simulink library "SendToSOMANET"  (R2016b)
settings: Solver=VariableStepAuto  StartTime=0.0  StopTime=10.0  RelTol=1e-3
undefined symbols (not defined in the file): jointPolarityLHFE, jointPolarityLKFE, jointPolarityRHFE, jointPolarityRKFE, resolutionJointEncoder, torquePolarityLHFE, torquePolarityLKFE, torquePolarityRHFE, torquePolarityRKFE, zeroOffsetLHFE, zeroOffsetLKFE, zeroOffsetRHFE, zeroOffsetRKFE
libraries: xpcethercatlib x35, ConversionsLibrary x32, simulink_extras x8
settings Model: Creator=Nathan  LastModifiedBy=march

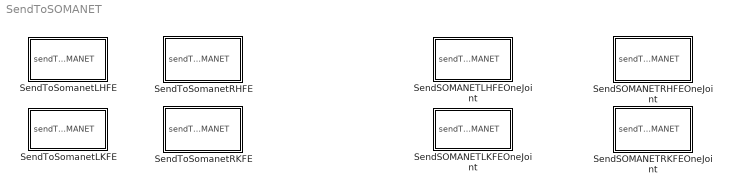
== system SendToSOMANET ==
  SendSOMANETLHFEOneJoint : Subsystem
  SendSOMANETLKFEOneJoint : Subsystem
  SendSOMANETRHFEOneJoint : Subsystem
  SendSOMANETRKFEOneJoint : Subsystem
  SendToSomanetLHFE : Subsystem
  SendToSomanetLKFE : Subsystem
  SendToSomanetRHFE : Subsystem
  SendToSomanetRKFE : Subsystem

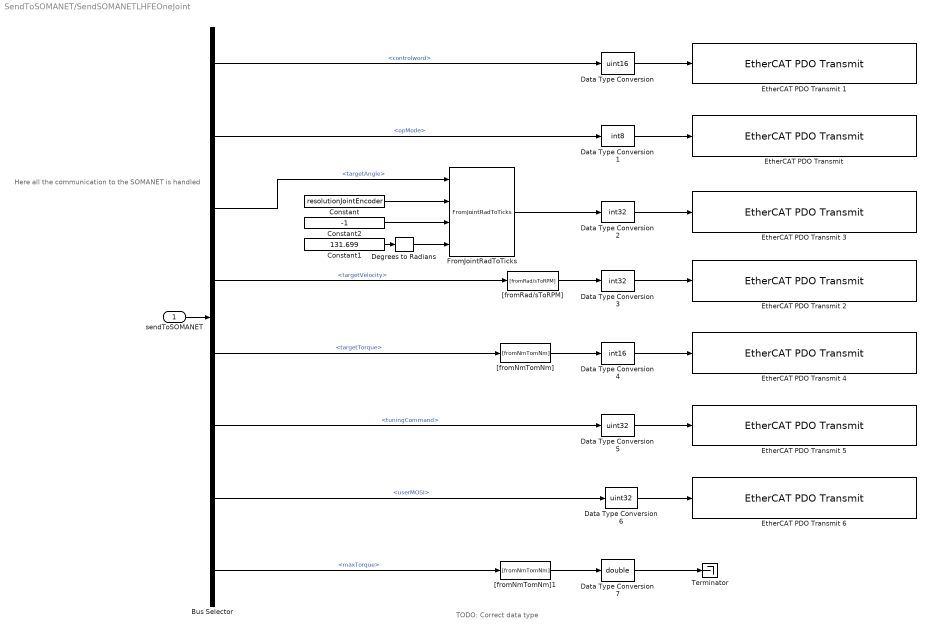
== system SendToSOMANET/SendSOMANETLHFEOneJoint ==
  note: Here all the communication to the SOMANET is handled
  note: TODO: Correct data type
  sendToSOMANET : Inport  OutDataTypeStr=Bus: EtherCATSendToSOMANET  BusOutputAsStruct=on
  Bus Selector : BusSelector  OutputSignals=controlword,opMode,targetAngle,targetVelocity,targetTorque,tuningCommand,userMOSI,maxTorque
  Constant : Constant  Value=resolutionJointEncoder
  Constant1 : Constant  Value=131.699  SampleTime=-1
  Constant2 : Constant  Value=-1
  Data Type Conversion : DataTypeConversion  OutDataTypeStr=uint16  RndMeth=Nearest
  Data Type Conversion1 : DataTypeConversion  OutDataTypeStr=int8  RndMeth=Nearest
  Data Type Conversion2 : DataTypeConversion  OutDataTypeStr=int32  RndMeth=Nearest
  Data Type Conversion3 : DataTypeConversion  OutDataTypeStr=int32  RndMeth=Nearest
  Data Type Conversion4 : DataTypeConversion  OutDataTypeStr=int16  RndMeth=Nearest
  Data Type Conversion5 : DataTypeConversion  OutDataTypeStr=uint32  RndMeth=Nearest
  Data Type Conversion6 : DataTypeConversion  OutDataTypeStr=uint32  RndMeth=Nearest
  Data Type Conversion7 : DataTypeConversion  OutDataTypeStr=double  RndMeth=Nearest
  Degrees to Radians : simulink_extras/Transformations/Degrees to Radians
  "EtherCAT PDO Transmit " : xpcethercatlib/EtherCAT PDO Transmit   Priority=3  sig_name=Drive 1 LHFE.Outputs.Op Mode  sig_offset=224  sig_type=int8  type_size=8  sig_dim=1  device_id=0  sample_time=0.002000
  EtherCAT PDO Transmit 1 : xpcethercatlib/EtherCAT PDO Transmit   Priority=3  sig_name=Drive 1 LHFE.Outputs.Controlword  sig_offset=208  sig_type=uint16  type_size=16  sig_dim=1  device_id=0  sample_time=0.002000
  EtherCAT PDO Transmit 2 : xpcethercatlib/EtherCAT PDO Transmit   Priority=3  sig_name=Drive 1 LHFE.Outputs.Target Velocity  sig_offset=280  sig_type=int32  type_size=32  sig_dim=1  device_id=0  sample_time=0.002000
  EtherCAT PDO Transmit 3 : xpcethercatlib/EtherCAT PDO Transmit   Priority=3  sig_name=Drive 1 LHFE.Outputs.Target Position  sig_offset=248  sig_type=int32  type_size=32  sig_dim=1  device_id=0  sample_time=0.002000
  EtherCAT PDO Transmit 4 : xpcethercatlib/EtherCAT PDO Transmit   Priority=3  sig_name=Drive 1 LHFE.Outputs.Target Torque  sig_offset=232  sig_type=int16  type_size=16  sig_dim=1  device_id=0  sample_time=0.002000
  EtherCAT PDO Transmit 5 : xpcethercatlib/EtherCAT PDO Transmit   Priority=3  sig_name=Drive 1 LHFE.Outputs.Tuning command  sig_offset=344  sig_type=uint32  type_size=32  sig_dim=1  device_id=0  sample_time=0.002000
  EtherCAT PDO Transmit 6 : xpcethercatlib/EtherCAT PDO Transmit   Priority=3  sig_name=Drive 1 LHFE.Outputs.User MOSI  sig_offset=408  sig_type=uint32  type_size=32  sig_dim=1  device_id=0  sample_time=0.002000
  FromJointRadToTicks : ConversionsLibrary/FromJointRadToTicks
  Terminator : Terminator
  "[fromNmTomNm]" : ConversionsLibrary/[fromNmTomNm]
  "[fromNmTomNm]1" : ConversionsLibrary/[fromNmTomNm]
  "[fromRad/sToRPM]" : ConversionsLibrary/[fromRad//sToRPM]
  wires:
  Bus Selector/1 -> Data Type Conversion/1  "<controlword>"
  "[fromRad/sToRPM]"/1 -> Data Type Conversion3/1
  Bus Selector/7 -> Data Type Conversion6/1  "<userMOSI>"
  Bus Selector/8 -> "[fromNmTomNm]1"/1  "<maxTorque>"
  Bus Selector/4 -> "[fromRad/sToRPM]"/1  "<targetVelocity>"
  "[fromNmTomNm]1"/1 -> Data Type Conversion7/1
  "[fromNmTomNm]"/1 -> Data Type Conversion4/1
  Bus Selector/6 -> Data Type Conversion5/1  "<tuningCommand>"
  Bus Selector/2 -> Data Type Conversion1/1  "<opMode>"
  Bus Selector/5 -> "[fromNmTomNm]"/1  "<targetTorque>"
  Data Type Conversion/1 -> EtherCAT PDO Transmit 1/1
  Data Type Conversion4/1 -> EtherCAT PDO Transmit 4/1
  Data Type Conversion3/1 -> EtherCAT PDO Transmit 2/1
  Data Type Conversion2/1 -> EtherCAT PDO Transmit 3/1
  Data Type Conversion1/1 -> "EtherCAT PDO Transmit "/1
  Data Type Conversion5/1 -> EtherCAT PDO Transmit 5/1
  Data Type Conversion6/1 -> EtherCAT PDO Transmit 6/1
  Data Type Conversion7/1 -> Terminator/1
  sendToSOMANET/1 -> Bus Selector/1
  Constant1/1 -> Degrees to Radians/1
  Bus Selector/3 -> FromJointRadToTicks/1  "<targetAngle>"
  Degrees to Radians/1 -> FromJointRadToTicks/4
  Constant/1 -> FromJointRadToTicks/2
  Constant2/1 -> FromJointRadToTicks/3
  FromJointRadToTicks/1 -> Data Type Conversion2/1

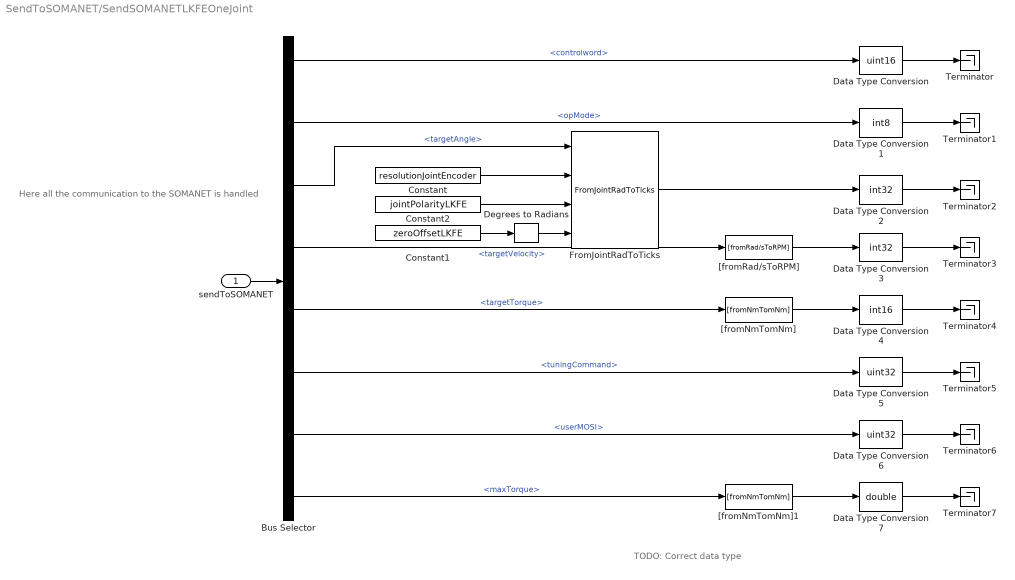
== system SendToSOMANET/SendSOMANETLKFEOneJoint ==
  note: Here all the communication to the SOMANET is handled
  note: TODO: Correct data type
  sendToSOMANET : Inport  OutDataTypeStr=Bus: EtherCATSendToSOMANET  BusOutputAsStruct=on
  Bus Selector : BusSelector  OutputSignals=controlword,opMode,targetAngle,targetVelocity,targetTorque,tuningCommand,userMOSI,maxTorque
  Constant : Constant  Value=resolutionJointEncoder
  Constant1 : Constant  Value=zeroOffsetLKFE  SampleTime=-1
  Constant2 : Constant  Value=jointPolarityLKFE
  Data Type Conversion : DataTypeConversion  OutDataTypeStr=uint16  RndMeth=Nearest
  Data Type Conversion1 : DataTypeConversion  OutDataTypeStr=int8  RndMeth=Nearest
  Data Type Conversion2 : DataTypeConversion  OutDataTypeStr=int32  RndMeth=Nearest
  Data Type Conversion3 : DataTypeConversion  OutDataTypeStr=int32  RndMeth=Nearest
  Data Type Conversion4 : DataTypeConversion  OutDataTypeStr=int16  RndMeth=Nearest
  Data Type Conversion5 : DataTypeConversion  OutDataTypeStr=uint32  RndMeth=Nearest
  Data Type Conversion6 : DataTypeConversion  OutDataTypeStr=uint32  RndMeth=Nearest
  Data Type Conversion7 : DataTypeConversion  OutDataTypeStr=double  RndMeth=Nearest
  Degrees to Radians : simulink_extras/Transformations/Degrees to Radians
  FromJointRadToTicks : ConversionsLibrary/FromJointRadToTicks
  Terminator{,1..7} (8 alike) : Terminator
  "[fromNmTomNm]" : ConversionsLibrary/[fromNmTomNm]
  "[fromNmTomNm]1" : ConversionsLibrary/[fromNmTomNm]
  "[fromRad/sToRPM]" : ConversionsLibrary/[fromRad//sToRPM]
  wires:
  Bus Selector/1 -> Data Type Conversion/1  "<controlword>"
  "[fromRad/sToRPM]"/1 -> Data Type Conversion3/1
  Bus Selector/7 -> Data Type Conversion6/1  "<userMOSI>"
  Bus Selector/8 -> "[fromNmTomNm]1"/1  "<maxTorque>"
  "[fromNmTomNm]1"/1 -> Data Type Conversion7/1
  "[fromNmTomNm]"/1 -> Data Type Conversion4/1
  Bus Selector/6 -> Data Type Conversion5/1  "<tuningCommand>"
  Bus Selector/2 -> Data Type Conversion1/1  "<opMode>"
  sendToSOMANET/1 -> Bus Selector/1
  Bus Selector/5 -> "[fromNmTomNm]"/1  "<targetTorque>"
  Data Type Conversion/1 -> Terminator/1
  Data Type Conversion1/1 -> Terminator1/1
  Data Type Conversion2/1 -> Terminator2/1
  Data Type Conversion3/1 -> Terminator3/1
  Data Type Conversion4/1 -> Terminator4/1
  Data Type Conversion5/1 -> Terminator5/1
  Data Type Conversion6/1 -> Terminator6/1
  Data Type Conversion7/1 -> Terminator7/1
  Bus Selector/3 -> FromJointRadToTicks/1  "<targetAngle>"
  Constant/1 -> FromJointRadToTicks/2
  Constant2/1 -> FromJointRadToTicks/3
  FromJointRadToTicks/1 -> Data Type Conversion2/1
  Constant1/1 -> Degrees to Radians/1
  Degrees to Radians/1 -> FromJointRadToTicks/4
  Bus Selector/4 -> "[fromRad/sToRPM]"/1  "<targetVelocity>"

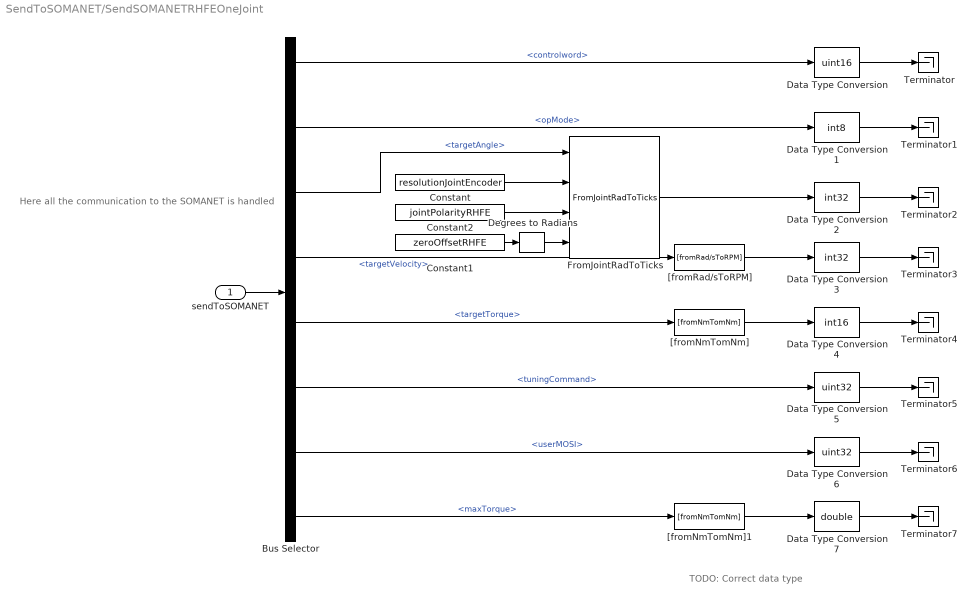
== system SendToSOMANET/SendSOMANETRHFEOneJoint ==
  note: Here all the communication to the SOMANET is handled
  note: TODO: Correct data type
  sendToSOMANET : Inport  OutDataTypeStr=Bus: EtherCATSendToSOMANET  BusOutputAsStruct=on
  Bus Selector : BusSelector  OutputSignals=controlword,opMode,targetAngle,targetVelocity,targetTorque,tuningCommand,userMOSI,maxTorque
  Constant : Constant  Value=resolutionJointEncoder
  Constant1 : Constant  Value=zeroOffsetRHFE  SampleTime=-1
  Constant2 : Constant  Value=jointPolarityRHFE
  Data Type Conversion : DataTypeConversion  OutDataTypeStr=uint16  RndMeth=Nearest
  Data Type Conversion1 : DataTypeConversion  OutDataTypeStr=int8  RndMeth=Nearest
  Data Type Conversion2 : DataTypeConversion  OutDataTypeStr=int32  RndMeth=Nearest
  Data Type Conversion3 : DataTypeConversion  OutDataTypeStr=int32  RndMeth=Nearest
  Data Type Conversion4 : DataTypeConversion  OutDataTypeStr=int16  RndMeth=Nearest
  Data Type Conversion5 : DataTypeConversion  OutDataTypeStr=uint32  RndMeth=Nearest
  Data Type Conversion6 : DataTypeConversion  OutDataTypeStr=uint32  RndMeth=Nearest
  Data Type Conversion7 : DataTypeConversion  OutDataTypeStr=double  RndMeth=Nearest
  Degrees to Radians : simulink_extras/Transformations/Degrees to Radians
  FromJointRadToTicks : ConversionsLibrary/FromJointRadToTicks
  Terminator{,1..7} (8 alike) : Terminator
  "[fromNmTomNm]" : ConversionsLibrary/[fromNmTomNm]
  "[fromNmTomNm]1" : ConversionsLibrary/[fromNmTomNm]
  "[fromRad/sToRPM]" : ConversionsLibrary/[fromRad//sToRPM]
  wires:
  Bus Selector/1 -> Data Type Conversion/1  "<controlword>"
  "[fromRad/sToRPM]"/1 -> Data Type Conversion3/1
  Bus Selector/7 -> Data Type Conversion6/1  "<userMOSI>"
  Bus Selector/8 -> "[fromNmTomNm]1"/1  "<maxTorque>"
  "[fromNmTomNm]1"/1 -> Data Type Conversion7/1
  "[fromNmTomNm]"/1 -> Data Type Conversion4/1
  Bus Selector/6 -> Data Type Conversion5/1  "<tuningCommand>"
  Bus Selector/2 -> Data Type Conversion1/1  "<opMode>"
  sendToSOMANET/1 -> Bus Selector/1
  Bus Selector/5 -> "[fromNmTomNm]"/1  "<targetTorque>"
  Data Type Conversion/1 -> Terminator/1
  Data Type Conversion1/1 -> Terminator1/1
  Data Type Conversion2/1 -> Terminator2/1
  Data Type Conversion3/1 -> Terminator3/1
  Data Type Conversion4/1 -> Terminator4/1
  Data Type Conversion5/1 -> Terminator5/1
  Data Type Conversion6/1 -> Terminator6/1
  Data Type Conversion7/1 -> Terminator7/1
  Bus Selector/3 -> FromJointRadToTicks/1  "<targetAngle>"
  Constant/1 -> FromJointRadToTicks/2
  Constant2/1 -> FromJointRadToTicks/3
  FromJointRadToTicks/1 -> Data Type Conversion2/1
  Constant1/1 -> Degrees to Radians/1
  Degrees to Radians/1 -> FromJointRadToTicks/4
  Bus Selector/4 -> "[fromRad/sToRPM]"/1  "<targetVelocity>"

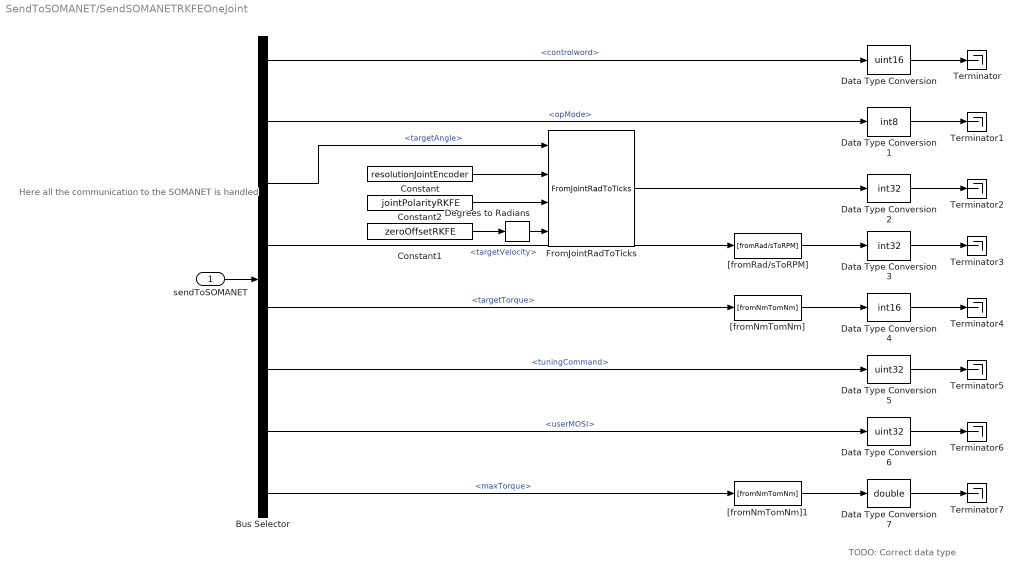
== system SendToSOMANET/SendSOMANETRKFEOneJoint ==
  note: Here all the communication to the SOMANET is handled
  note: TODO: Correct data type
  sendToSOMANET : Inport  OutDataTypeStr=Bus: EtherCATSendToSOMANET  BusOutputAsStruct=on
  Bus Selector : BusSelector  OutputSignals=controlword,opMode,targetAngle,targetVelocity,targetTorque,tuningCommand,userMOSI,maxTorque
  Constant : Constant  Value=resolutionJointEncoder
  Constant1 : Constant  Value=zeroOffsetRKFE  SampleTime=-1
  Constant2 : Constant  Value=jointPolarityRKFE
  Data Type Conversion : DataTypeConversion  OutDataTypeStr=uint16  RndMeth=Nearest
  Data Type Conversion1 : DataTypeConversion  OutDataTypeStr=int8  RndMeth=Nearest
  Data Type Conversion2 : DataTypeConversion  OutDataTypeStr=int32  RndMeth=Nearest
  Data Type Conversion3 : DataTypeConversion  OutDataTypeStr=int32  RndMeth=Nearest
  Data Type Conversion4 : DataTypeConversion  OutDataTypeStr=int16  RndMeth=Nearest
  Data Type Conversion5 : DataTypeConversion  OutDataTypeStr=uint32  RndMeth=Nearest
  Data Type Conversion6 : DataTypeConversion  OutDataTypeStr=uint32  RndMeth=Nearest
  Data Type Conversion7 : DataTypeConversion  OutDataTypeStr=double  RndMeth=Nearest
  Degrees to Radians : simulink_extras/Transformations/Degrees to Radians
  FromJointRadToTicks : ConversionsLibrary/FromJointRadToTicks
  Terminator{,1..7} (8 alike) : Terminator
  "[fromNmTomNm]" : ConversionsLibrary/[fromNmTomNm]
  "[fromNmTomNm]1" : ConversionsLibrary/[fromNmTomNm]
  "[fromRad/sToRPM]" : ConversionsLibrary/[fromRad//sToRPM]
  wires:
  Bus Selector/1 -> Data Type Conversion/1  "<controlword>"
  "[fromRad/sToRPM]"/1 -> Data Type Conversion3/1
  Bus Selector/7 -> Data Type Conversion6/1  "<userMOSI>"
  Bus Selector/8 -> "[fromNmTomNm]1"/1  "<maxTorque>"
  Bus Selector/4 -> "[fromRad/sToRPM]"/1  "<targetVelocity>"
  "[fromNmTomNm]1"/1 -> Data Type Conversion7/1
  "[fromNmTomNm]"/1 -> Data Type Conversion4/1
  Bus Selector/6 -> Data Type Conversion5/1  "<tuningCommand>"
  Bus Selector/2 -> Data Type Conversion1/1  "<opMode>"
  sendToSOMANET/1 -> Bus Selector/1
  Bus Selector/5 -> "[fromNmTomNm]"/1  "<targetTorque>"
  Data Type Conversion/1 -> Terminator/1
  Data Type Conversion1/1 -> Terminator1/1
  Data Type Conversion2/1 -> Terminator2/1
  Data Type Conversion3/1 -> Terminator3/1
  Data Type Conversion4/1 -> Terminator4/1
  Data Type Conversion5/1 -> Terminator5/1
  Data Type Conversion6/1 -> Terminator6/1
  Data Type Conversion7/1 -> Terminator7/1
  Constant1/1 -> Degrees to Radians/1
  Bus Selector/3 -> FromJointRadToTicks/1  "<targetAngle>"
  Degrees to Radians/1 -> FromJointRadToTicks/4
  Constant/1 -> FromJointRadToTicks/2
  Constant2/1 -> FromJointRadToTicks/3
  FromJointRadToTicks/1 -> Data Type Conversion2/1

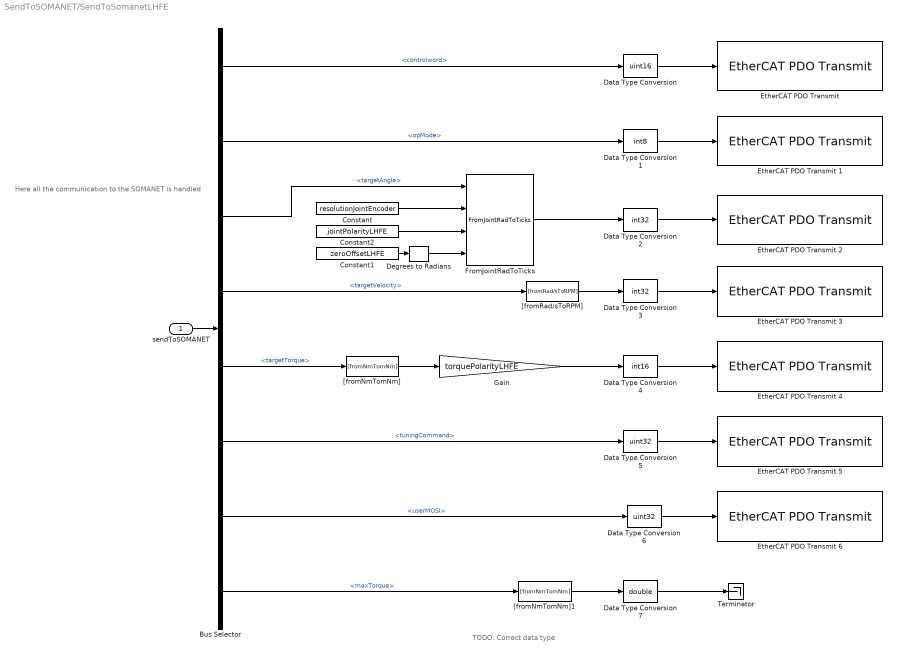
== system SendToSOMANET/SendToSomanetLHFE ==
  note: TODO: Correct data type
  note: Here all the communication to the SOMANET is handled
  sendToSOMANET : Inport  OutDataTypeStr=Bus: EtherCATSendToSOMANET  BusOutputAsStruct=on
  Bus Selector : BusSelector  OutputSignals=controlword,opMode,targetAngle,targetVelocity,targetTorque,tuningCommand,userMOSI,maxTorque
  Constant : Constant  Value=resolutionJointEncoder
  Constant1 : Constant  Value=zeroOffsetLHFE  SampleTime=-1
  Constant2 : Constant  Value=jointPolarityLHFE
  Data Type Conversion : DataTypeConversion  OutDataTypeStr=uint16  RndMeth=Nearest
  Data Type Conversion1 : DataTypeConversion  OutDataTypeStr=int8  RndMeth=Nearest
  Data Type Conversion2 : DataTypeConversion  OutDataTypeStr=int32  RndMeth=Nearest
  Data Type Conversion3 : DataTypeConversion  OutDataTypeStr=int32  RndMeth=Nearest
  Data Type Conversion4 : DataTypeConversion  OutDataTypeStr=int16  RndMeth=Nearest
  Data Type Conversion5 : DataTypeConversion  OutDataTypeStr=uint32  RndMeth=Nearest
  Data Type Conversion6 : DataTypeConversion  OutDataTypeStr=uint32  RndMeth=Nearest
  Data Type Conversion7 : DataTypeConversion  OutDataTypeStr=double  RndMeth=Nearest
  Degrees to Radians : simulink_extras/Transformations/Degrees to Radians
  "EtherCAT PDO Transmit " : xpcethercatlib/EtherCAT PDO Transmit   Priority=3  sig_name=Drive 1 LHFE.Outputs.Controlword  sig_offset=208  sig_type=uint16  type_size=16  sig_dim=1  device_id=0  sample_time=0.002000
  EtherCAT PDO Transmit 1 : xpcethercatlib/EtherCAT PDO Transmit   Priority=3  sig_name=Drive 1 LHFE.Outputs.Op Mode  sig_offset=224  sig_type=int8  type_size=8  sig_dim=1  device_id=0  sample_time=0.002000
  EtherCAT PDO Transmit 2 : xpcethercatlib/EtherCAT PDO Transmit   Priority=3  sig_name=Drive 1 LHFE.Outputs.Target Position  sig_offset=248  sig_type=int32  type_size=32  sig_dim=1  device_id=0  sample_time=0.002000
  EtherCAT PDO Transmit 3 : xpcethercatlib/EtherCAT PDO Transmit   Priority=3  sig_name=Drive 1 LHFE.Outputs.Target Velocity  sig_offset=280  sig_type=int32  type_size=32  sig_dim=1  device_id=0  sample_time=0.002000
  EtherCAT PDO Transmit 4 : xpcethercatlib/EtherCAT PDO Transmit   Priority=3  sig_name=Drive 1 LHFE.Outputs.Target Torque  sig_offset=232  sig_type=int16  type_size=16  sig_dim=1  device_id=0  sample_time=0.002000
  EtherCAT PDO Transmit 5 : xpcethercatlib/EtherCAT PDO Transmit   Priority=3  sig_name=Drive 1 LHFE.Outputs.Tuning command  sig_offset=344  sig_type=uint32  type_size=32  sig_dim=1  device_id=0  sample_time=0.002000
  EtherCAT PDO Transmit 6 : xpcethercatlib/EtherCAT PDO Transmit   Priority=3  sig_name=Drive 1 LHFE.Outputs.User MOSI  sig_offset=408  sig_type=uint32  type_size=32  sig_dim=1  device_id=0  sample_time=0.002000
  FromJointRadToTicks : ConversionsLibrary/FromJointRadToTicks
  Gain : Gain  Gain=torquePolarityLHFE
  Terminator : Terminator
  "[fromNmTomNm]" : ConversionsLibrary/[fromNmTomNm]
  "[fromNmTomNm]1" : ConversionsLibrary/[fromNmTomNm]
  "[fromRad/sToRPM]" : ConversionsLibrary/[fromRad//sToRPM]
  wires:
  sendToSOMANET/1 -> Bus Selector/1
  Data Type Conversion7/1 -> Terminator/1
  Data Type Conversion6/1 -> EtherCAT PDO Transmit 6/1
  Data Type Conversion5/1 -> EtherCAT PDO Transmit 5/1
  Data Type Conversion1/1 -> EtherCAT PDO Transmit 1/1
  Data Type Conversion2/1 -> EtherCAT PDO Transmit 2/1
  Data Type Conversion3/1 -> EtherCAT PDO Transmit 3/1
  Data Type Conversion4/1 -> EtherCAT PDO Transmit 4/1
  Data Type Conversion/1 -> "EtherCAT PDO Transmit "/1
  Bus Selector/5 -> "[fromNmTomNm]"/1  "<targetTorque>"
  Bus Selector/2 -> Data Type Conversion1/1  "<opMode>"
  Bus Selector/6 -> Data Type Conversion5/1  "<tuningCommand>"
  "[fromNmTomNm]"/1 -> Gain/1
  "[fromNmTomNm]1"/1 -> Data Type Conversion7/1
  Bus Selector/4 -> "[fromRad/sToRPM]"/1  "<targetVelocity>"
  Bus Selector/8 -> "[fromNmTomNm]1"/1  "<maxTorque>"
  Bus Selector/7 -> Data Type Conversion6/1  "<userMOSI>"
  "[fromRad/sToRPM]"/1 -> Data Type Conversion3/1
  Bus Selector/1 -> Data Type Conversion/1  "<controlword>"
  Constant1/1 -> Degrees to Radians/1
  Bus Selector/3 -> FromJointRadToTicks/1  "<targetAngle>"
  Degrees to Radians/1 -> FromJointRadToTicks/4
  Constant/1 -> FromJointRadToTicks/2
  Constant2/1 -> FromJointRadToTicks/3
  FromJointRadToTicks/1 -> Data Type Conversion2/1
  Gain/1 -> Data Type Conversion4/1

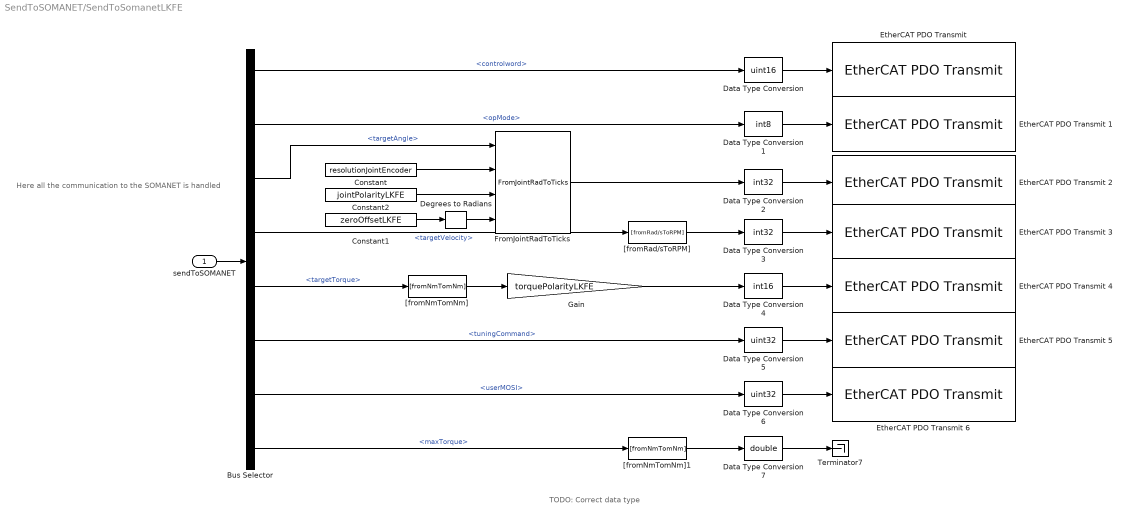
== system SendToSOMANET/SendToSomanetLKFE ==
  note: TODO: Correct data type
  note: Here all the communication to the SOMANET is handled
  sendToSOMANET : Inport  OutDataTypeStr=Bus: EtherCATSendToSOMANET  BusOutputAsStruct=on
  Bus Selector : BusSelector  OutputSignals=controlword,opMode,targetAngle,targetVelocity,targetTorque,tuningCommand,userMOSI,maxTorque
  Constant : Constant  Value=resolutionJointEncoder
  Constant1 : Constant  Value=zeroOffsetLKFE  SampleTime=-1
  Constant2 : Constant  Value=jointPolarityLKFE
  Data Type Conversion : DataTypeConversion  OutDataTypeStr=uint16  RndMeth=Nearest
  Data Type Conversion1 : DataTypeConversion  OutDataTypeStr=int8  RndMeth=Nearest
  Data Type Conversion2 : DataTypeConversion  OutDataTypeStr=int32  RndMeth=Nearest
  Data Type Conversion3 : DataTypeConversion  OutDataTypeStr=int32  RndMeth=Nearest
  Data Type Conversion4 : DataTypeConversion  OutDataTypeStr=int16  RndMeth=Nearest
  Data Type Conversion5 : DataTypeConversion  OutDataTypeStr=uint32  RndMeth=Nearest
  Data Type Conversion6 : DataTypeConversion  OutDataTypeStr=uint32  RndMeth=Nearest
  Data Type Conversion7 : DataTypeConversion  OutDataTypeStr=double  RndMeth=Nearest
  Degrees to Radians : simulink_extras/Transformations/Degrees to Radians
  "EtherCAT PDO Transmit " : xpcethercatlib/EtherCAT PDO Transmit   Priority=3  sig_name=Drive 2 LKFE.Outputs.Controlword  sig_offset=632  sig_type=uint16  type_size=16  sig_dim=1  device_id=0  sample_time=0.002000
  EtherCAT PDO Transmit 1 : xpcethercatlib/EtherCAT PDO Transmit   Priority=3  sig_name=Drive 2 LKFE.Outputs.Op Mode  sig_offset=648  sig_type=int8  type_size=8  sig_dim=1  device_id=0  sample_time=0.002000
  EtherCAT PDO Transmit 2 : xpcethercatlib/EtherCAT PDO Transmit   Priority=3  sig_name=Drive 2 LKFE.Outputs.Target Position  sig_offset=672  sig_type=int32  type_size=32  sig_dim=1  device_id=0  sample_time=0.002000
  EtherCAT PDO Transmit 3 : xpcethercatlib/EtherCAT PDO Transmit   Priority=3  sig_name=Drive 2 LKFE.Outputs.Target Velocity  sig_offset=704  sig_type=int32  type_size=32  sig_dim=1  device_id=0  sample_time=0.002000
  EtherCAT PDO Transmit 4 : xpcethercatlib/EtherCAT PDO Transmit   Priority=3  sig_name=Drive 2 LKFE.Outputs.Target Torque  sig_offset=656  sig_type=int16  type_size=16  sig_dim=1  device_id=0  sample_time=0.002000
  EtherCAT PDO Transmit 5 : xpcethercatlib/EtherCAT PDO Transmit   Priority=3  sig_name=Drive 2 LKFE.Outputs.Tuning command  sig_offset=768  sig_type=uint32  type_size=32  sig_dim=1  device_id=0  sample_time=0.002000
  EtherCAT PDO Transmit 6 : xpcethercatlib/EtherCAT PDO Transmit   Priority=3  sig_name=Drive 2 LKFE.Outputs.User MOSI  sig_offset=832  sig_type=uint32  type_size=32  sig_dim=1  device_id=0  sample_time=0.002000
  FromJointRadToTicks : ConversionsLibrary/FromJointRadToTicks
  Gain : Gain  Gain=torquePolarityLKFE
  Terminator7 : Terminator
  "[fromNmTomNm]" : ConversionsLibrary/[fromNmTomNm]
  "[fromNmTomNm]1" : ConversionsLibrary/[fromNmTomNm]
  "[fromRad/sToRPM]" : ConversionsLibrary/[fromRad//sToRPM]
  wires:
  Data Type Conversion7/1 -> Terminator7/1
  Data Type Conversion6/1 -> EtherCAT PDO Transmit 6/1
  Data Type Conversion5/1 -> EtherCAT PDO Transmit 5/1
  Data Type Conversion4/1 -> EtherCAT PDO Transmit 4/1
  Data Type Conversion3/1 -> EtherCAT PDO Transmit 3/1
  Data Type Conversion2/1 -> EtherCAT PDO Transmit 2/1
  Data Type Conversion1/1 -> EtherCAT PDO Transmit 1/1
  Data Type Conversion/1 -> "EtherCAT PDO Transmit "/1
  Bus Selector/5 -> "[fromNmTomNm]"/1  "<targetTorque>"
  sendToSOMANET/1 -> Bus Selector/1
  Bus Selector/2 -> Data Type Conversion1/1  "<opMode>"
  Bus Selector/6 -> Data Type Conversion5/1  "<tuningCommand>"
  "[fromNmTomNm]"/1 -> Gain/1
  "[fromNmTomNm]1"/1 -> Data Type Conversion7/1
  Bus Selector/4 -> "[fromRad/sToRPM]"/1  "<targetVelocity>"
  Bus Selector/8 -> "[fromNmTomNm]1"/1  "<maxTorque>"
  Bus Selector/7 -> Data Type Conversion6/1  "<userMOSI>"
  "[fromRad/sToRPM]"/1 -> Data Type Conversion3/1
  Bus Selector/1 -> Data Type Conversion/1  "<controlword>"
  Constant1/1 -> Degrees to Radians/1
  Bus Selector/3 -> FromJointRadToTicks/1  "<targetAngle>"
  Degrees to Radians/1 -> FromJointRadToTicks/4
  Constant/1 -> FromJointRadToTicks/2
  Constant2/1 -> FromJointRadToTicks/3
  FromJointRadToTicks/1 -> Data Type Conversion2/1
  Gain/1 -> Data Type Conversion4/1

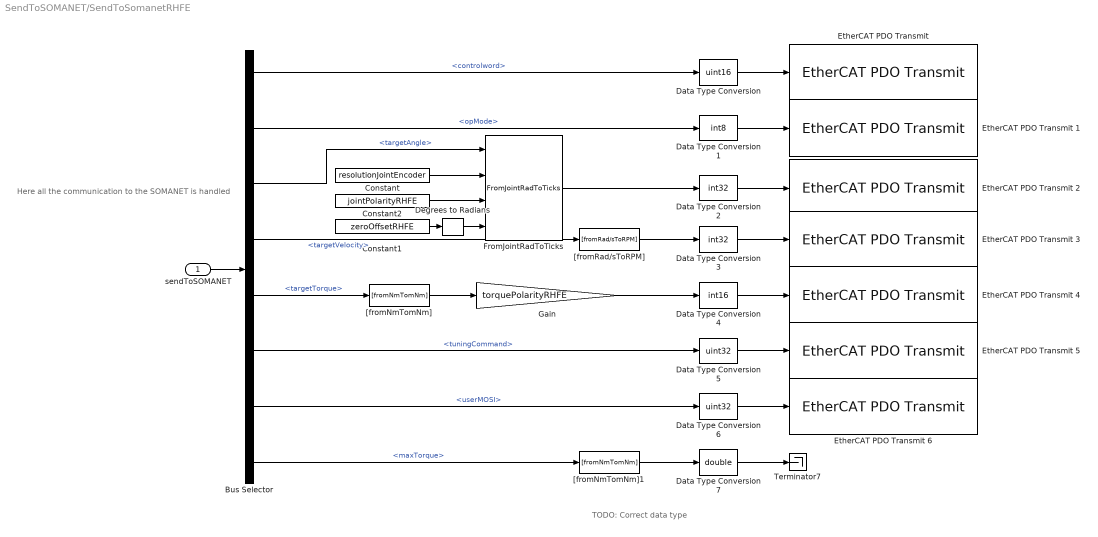
== system SendToSOMANET/SendToSomanetRHFE ==
  note: TODO: Correct data type
  note: Here all the communication to the SOMANET is handled
  sendToSOMANET : Inport  OutDataTypeStr=Bus: EtherCATSendToSOMANET  BusOutputAsStruct=on
  Bus Selector : BusSelector  OutputSignals=controlword,opMode,targetAngle,targetVelocity,targetTorque,tuningCommand,userMOSI,maxTorque
  Constant : Constant  Value=resolutionJointEncoder
  Constant1 : Constant  Value=zeroOffsetRHFE  SampleTime=-1
  Constant2 : Constant  Value=jointPolarityRHFE
  Data Type Conversion : DataTypeConversion  OutDataTypeStr=uint16  RndMeth=Nearest
  Data Type Conversion1 : DataTypeConversion  OutDataTypeStr=int8  RndMeth=Nearest
  Data Type Conversion2 : DataTypeConversion  OutDataTypeStr=int32  RndMeth=Nearest
  Data Type Conversion3 : DataTypeConversion  OutDataTypeStr=int32  RndMeth=Nearest
  Data Type Conversion4 : DataTypeConversion  OutDataTypeStr=int16  RndMeth=Nearest
  Data Type Conversion5 : DataTypeConversion  OutDataTypeStr=uint32  RndMeth=Nearest
  Data Type Conversion6 : DataTypeConversion  OutDataTypeStr=uint32  RndMeth=Nearest
  Data Type Conversion7 : DataTypeConversion  OutDataTypeStr=double  RndMeth=Nearest
  Degrees to Radians : simulink_extras/Transformations/Degrees to Radians
  "EtherCAT PDO Transmit " : xpcethercatlib/EtherCAT PDO Transmit   Priority=3  sig_name=Drive 3 RHFE.Outputs.Controlword  sig_offset=1056  sig_type=uint16  type_size=16  sig_dim=1  device_id=0  sample_time=0.002000
  EtherCAT PDO Transmit 1 : xpcethercatlib/EtherCAT PDO Transmit   Priority=3  sig_name=Drive 3 RHFE.Outputs.Op Mode  sig_offset=1072  sig_type=int8  type_size=8  sig_dim=1  device_id=0  sample_time=0.002000
  EtherCAT PDO Transmit 2 : xpcethercatlib/EtherCAT PDO Transmit   Priority=3  sig_name=Drive 3 RHFE.Outputs.Target Position  sig_offset=1096  sig_type=int32  type_size=32  sig_dim=1  device_id=0  sample_time=0.002000
  EtherCAT PDO Transmit 3 : xpcethercatlib/EtherCAT PDO Transmit   Priority=3  sig_name=Drive 3 RHFE.Outputs.Target Velocity  sig_offset=1128  sig_type=int32  type_size=32  sig_dim=1  device_id=0  sample_time=0.002000
  EtherCAT PDO Transmit 4 : xpcethercatlib/EtherCAT PDO Transmit   Priority=3  sig_name=Drive 3 RHFE.Outputs.Target Torque  sig_offset=1080  sig_type=int16  type_size=16  sig_dim=1  device_id=0  sample_time=0.002000
  EtherCAT PDO Transmit 5 : xpcethercatlib/EtherCAT PDO Transmit   Priority=3  sig_name=Drive 3 RHFE.Outputs.Tuning command  sig_offset=1192  sig_type=uint32  type_size=32  sig_dim=1  device_id=0  sample_time=0.002000
  EtherCAT PDO Transmit 6 : xpcethercatlib/EtherCAT PDO Transmit   Priority=3  sig_name=Drive 3 RHFE.Outputs.User MOSI  sig_offset=1256  sig_type=uint32  type_size=32  sig_dim=1  device_id=0  sample_time=0.002000
  FromJointRadToTicks : ConversionsLibrary/FromJointRadToTicks
  Gain : Gain  Gain=torquePolarityRHFE
  Terminator7 : Terminator
  "[fromNmTomNm]" : ConversionsLibrary/[fromNmTomNm]
  "[fromNmTomNm]1" : ConversionsLibrary/[fromNmTomNm]
  "[fromRad/sToRPM]" : ConversionsLibrary/[fromRad//sToRPM]
  wires:
  Data Type Conversion7/1 -> Terminator7/1
  Data Type Conversion6/1 -> EtherCAT PDO Transmit 6/1
  Data Type Conversion5/1 -> EtherCAT PDO Transmit 5/1
  Data Type Conversion4/1 -> EtherCAT PDO Transmit 4/1
  Data Type Conversion3/1 -> EtherCAT PDO Transmit 3/1
  Data Type Conversion2/1 -> EtherCAT PDO Transmit 2/1
  Data Type Conversion1/1 -> EtherCAT PDO Transmit 1/1
  Data Type Conversion/1 -> "EtherCAT PDO Transmit "/1
  Bus Selector/5 -> "[fromNmTomNm]"/1  "<targetTorque>"
  sendToSOMANET/1 -> Bus Selector/1
  Bus Selector/2 -> Data Type Conversion1/1  "<opMode>"
  Bus Selector/6 -> Data Type Conversion5/1  "<tuningCommand>"
  "[fromNmTomNm]"/1 -> Gain/1
  "[fromNmTomNm]1"/1 -> Data Type Conversion7/1
  Bus Selector/4 -> "[fromRad/sToRPM]"/1  "<targetVelocity>"
  Bus Selector/8 -> "[fromNmTomNm]1"/1  "<maxTorque>"
  Bus Selector/7 -> Data Type Conversion6/1  "<userMOSI>"
  "[fromRad/sToRPM]"/1 -> Data Type Conversion3/1
  Bus Selector/1 -> Data Type Conversion/1  "<controlword>"
  Constant1/1 -> Degrees to Radians/1
  Bus Selector/3 -> FromJointRadToTicks/1  "<targetAngle>"
  Degrees to Radians/1 -> FromJointRadToTicks/4
  Constant/1 -> FromJointRadToTicks/2
  Constant2/1 -> FromJointRadToTicks/3
  FromJointRadToTicks/1 -> Data Type Conversion2/1
  Gain/1 -> Data Type Conversion4/1

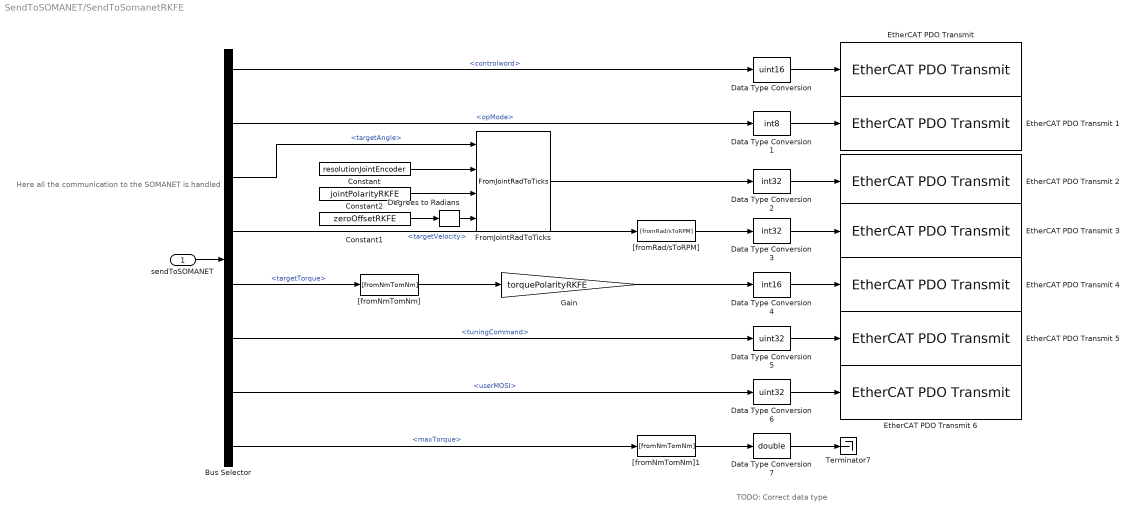
== system SendToSOMANET/SendToSomanetRKFE ==
  note: TODO: Correct data type
  note: Here all the communication to the SOMANET is handled
  sendToSOMANET : Inport  OutDataTypeStr=Bus: EtherCATSendToSOMANET  BusOutputAsStruct=on
  Bus Selector : BusSelector  OutputSignals=controlword,opMode,targetAngle,targetVelocity,targetTorque,tuningCommand,userMOSI,maxTorque
  Constant : Constant  Value=resolutionJointEncoder
  Constant1 : Constant  Value=zeroOffsetRKFE  SampleTime=-1
  Constant2 : Constant  Value=jointPolarityRKFE
  Data Type Conversion : DataTypeConversion  OutDataTypeStr=uint16  RndMeth=Nearest
  Data Type Conversion1 : DataTypeConversion  OutDataTypeStr=int8  RndMeth=Nearest
  Data Type Conversion2 : DataTypeConversion  OutDataTypeStr=int32  RndMeth=Nearest
  Data Type Conversion3 : DataTypeConversion  OutDataTypeStr=int32  RndMeth=Nearest
  Data Type Conversion4 : DataTypeConversion  OutDataTypeStr=int16  RndMeth=Nearest
  Data Type Conversion5 : DataTypeConversion  OutDataTypeStr=uint32  RndMeth=Nearest
  Data Type Conversion6 : DataTypeConversion  OutDataTypeStr=uint32  RndMeth=Nearest
  Data Type Conversion7 : DataTypeConversion  OutDataTypeStr=double  RndMeth=Nearest
  Degrees to Radians : simulink_extras/Transformations/Degrees to Radians
  "EtherCAT PDO Transmit " : xpcethercatlib/EtherCAT PDO Transmit   Priority=3  sig_name=Drive 4 RKFE.Outputs.Controlword  sig_offset=1480  sig_type=uint16  type_size=16  sig_dim=1  device_id=0  sample_time=0.002000
  EtherCAT PDO Transmit 1 : xpcethercatlib/EtherCAT PDO Transmit   Priority=3  sig_name=Drive 4 RKFE.Outputs.Op Mode  sig_offset=1496  sig_type=int8  type_size=8  sig_dim=1  device_id=0  sample_time=0.002000
  EtherCAT PDO Transmit 2 : xpcethercatlib/EtherCAT PDO Transmit   Priority=3  sig_name=Drive 4 RKFE.Outputs.Target Position  sig_offset=1520  sig_type=int32  type_size=32  sig_dim=1  device_id=0  sample_time=0.002000
  EtherCAT PDO Transmit 3 : xpcethercatlib/EtherCAT PDO Transmit   Priority=3  sig_name=Drive 4 RKFE.Outputs.Target Velocity  sig_offset=1552  sig_type=int32  type_size=32  sig_dim=1  device_id=0  sample_time=0.002000
  EtherCAT PDO Transmit 4 : xpcethercatlib/EtherCAT PDO Transmit   Priority=3  sig_name=Drive 4 RKFE.Outputs.Target Torque  sig_offset=1504  sig_type=int16  type_size=16  sig_dim=1  device_id=0  sample_time=0.002000
  EtherCAT PDO Transmit 5 : xpcethercatlib/EtherCAT PDO Transmit   Priority=3  sig_name=Drive 4 RKFE.Outputs.Tuning command  sig_offset=1616  sig_type=uint32  type_size=32  sig_dim=1  device_id=0  sample_time=0.002000
  EtherCAT PDO Transmit 6 : xpcethercatlib/EtherCAT PDO Transmit   Priority=3  sig_name=Drive 4 RKFE.Outputs.User MOSI  sig_offset=1680  sig_type=uint32  type_size=32  sig_dim=1  device_id=0  sample_time=0.002000
  FromJointRadToTicks : ConversionsLibrary/FromJointRadToTicks
  Gain : Gain  Gain=torquePolarityRKFE
  Terminator7 : Terminator
  "[fromNmTomNm]" : ConversionsLibrary/[fromNmTomNm]
  "[fromNmTomNm]1" : ConversionsLibrary/[fromNmTomNm]
  "[fromRad/sToRPM]" : ConversionsLibrary/[fromRad//sToRPM]
  wires:
  Data Type Conversion7/1 -> Terminator7/1
  Data Type Conversion6/1 -> EtherCAT PDO Transmit 6/1
  Data Type Conversion5/1 -> EtherCAT PDO Transmit 5/1
  Data Type Conversion4/1 -> EtherCAT PDO Transmit 4/1
  Data Type Conversion3/1 -> EtherCAT PDO Transmit 3/1
  Data Type Conversion2/1 -> EtherCAT PDO Transmit 2/1
  Data Type Conversion1/1 -> EtherCAT PDO Transmit 1/1
  Data Type Conversion/1 -> "EtherCAT PDO Transmit "/1
  Bus Selector/5 -> "[fromNmTomNm]"/1  "<targetTorque>"
  sendToSOMANET/1 -> Bus Selector/1
  Bus Selector/2 -> Data Type Conversion1/1  "<opMode>"
  Bus Selector/6 -> Data Type Conversion5/1  "<tuningCommand>"
  "[fromNmTomNm]"/1 -> Gain/1
  "[fromNmTomNm]1"/1 -> Data Type Conversion7/1
  Bus Selector/4 -> "[fromRad/sToRPM]"/1  "<targetVelocity>"
  Bus Selector/8 -> "[fromNmTomNm]1"/1  "<maxTorque>"
  Bus Selector/7 -> Data Type Conversion6/1  "<userMOSI>"
  "[fromRad/sToRPM]"/1 -> Data Type Conversion3/1
  Bus Selector/1 -> Data Type Conversion/1  "<controlword>"
  Constant1/1 -> Degrees to Radians/1
  Bus Selector/3 -> FromJointRadToTicks/1  "<targetAngle>"
  Degrees to Radians/1 -> FromJointRadToTicks/4
  Constant/1 -> FromJointRadToTicks/2
  Constant2/1 -> FromJointRadToTicks/3
  FromJointRadToTicks/1 -> Data Type Conversion2/1
  Gain/1 -> Data Type Conversion4/1
